simulink subsystem "StatePropagation"  (R2022a)
settings: Solver=VariableStepAuto  StartTime=0.0  StopTime=10.0  RelTol=1e-3
model mask{spaceRobot=spaceRobot}
settings Model: Creator=charl  LastModifiedBy=charl

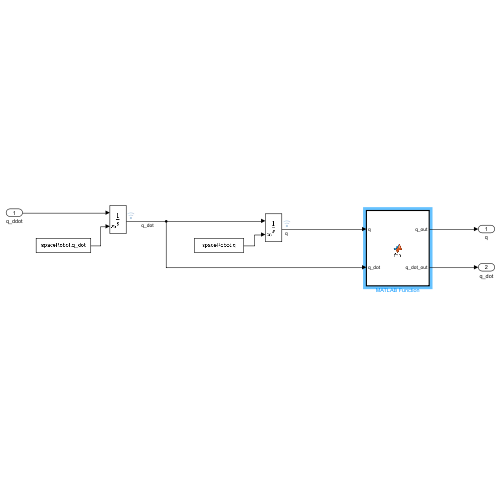
[thumbnail: Simulink's stored preview of the top-level diagram]
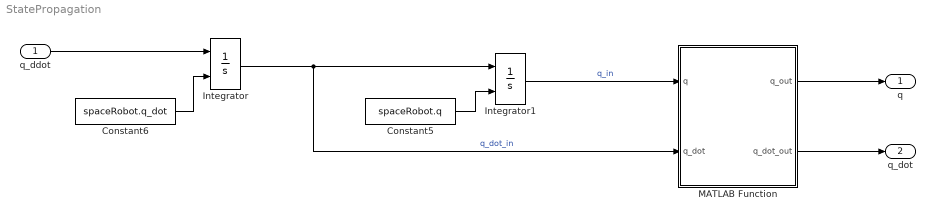
== system StatePropagation ==
  q_ddot : Inport
  Constant5 : Constant  Value=spaceRobot.q
  Constant6 : Constant  Value=spaceRobot.q_dot
  Integrator : Integrator  InitialConditionSource=external
  Integrator1 : Integrator  InitialConditionSource=external
  MATLAB Function : MATLAB Function  TreatAsAtomicUnit=on
  q : Outport
  q_dot : Outport  Port=2
  wires:
  MATLAB Function/2(q_dot_out) -> q_dot/1
  MATLAB Function/1(q_out) -> q/1
  q_ddot/1 -> Integrator/1
  Constant6/1 -> Integrator/2
  Integrator/1 -> Integrator1/1, MATLAB Function/2(q_dot)  "q_dot_in"
  Constant5/1 -> Integrator1/2
  Integrator1/1 -> MATLAB Function/1(q)  "q_in"

== matlab function StatePropagation/MATLAB Function ==
  data: q input; q_out output; q_dot input; q_dot_out output; jointLims parameter
function [q_out, q_dot_out] = fcn(q, q_dot, jointLims)

q_out = q;  
q_dot_out = q_dot;

for i=7:6+size(jointLims, 1)
    lims = jointLims(i-6, :);


    if q(i) < lims(1)
        q_out(i) = lims(1);
        q_dot_out(i) = 0;

    elseif q(i) > lims(2)
        q_out(i) = lims(2);
        q_dot_out(i) = 0;
    end
end
